simulink model "TorqueVect"  (R2022a)
settings: Solver=VariableStepAuto  StartTime=0.0  StopTime=32  RelTol=1e-3
PreLoadFcn:
  | run('Parameters\FSE_Parameters.m')
undefined symbols (not defined in the file): BRegenEnabledButton, canChannel, CyalphaLookUp, efficiency, Fz_curve, Fz_scaling_long, gearR, izz, jw, Kd, kd, Ki, ki, Kp, kp, l_f, l_r, lambda, m, Mz_max, N, N_lat, N_long, P_max, pid_kd_lat, pid_kd_long, pid_ki_lat, pid_ki_long, pid_kp_lat, pid_kp_long, R_max, rw, steerR, T_i_max, TC_Decr_Gas, TC_Derivative, TC_Incr_Gas, TC_On, TC_Relay_Off, TC_Relay_On, tireCornerStiffness, Ts, TV_On, TV_Override, velocity_lookup, velocity_lookup_lat, y_ref, yrr_scaling
libraries: simulink x218, slpidlib x135, CarMaker4SL x101, TractionControlLibrary x13, canmsglib x9, canlib x8, TorqueVectoringLibrary x6, simulink_extras x4, PedalConversionLibrary x3, PowerControlLibrary x1
(part 12 of 26)

== system TorqueVect/CarMaker/IPG Vehicle/PowerTrain/PTControl Example/PTControl_TV_MFE2/New TC/TC R2 ==
  modified slip ratio reference : Inport
  lim 1 : Inport  Port=2
  modified slip ratio measurement : Inport  Port=3
  P_TC : Inport  Port=4
  D_TC : Inport  Port=5
  enable_tc : Inport  Port=6
  PID Controller : slpidlib/PID Controller  Commented=on  Controller=PD  Form=Parallel  TimeDomain=Discrete-time  UseExternalTs=off  SampleTime=-1  IntegratorMethod=Forward Euler  FilterMethod=Forward Euler  ControllerParametersSource=external  P=125  I=1  UseKiTs=on  D=0  N=100  UseFilter=on  TunerSelectOption=Transfer Function Based (PID Tuner App)  InitialConditionSource=internal  InitialConditionForIntegrator=0  InitialConditionForFilter=0  DifferentiatorICPrevScaledInput=0  ExternalReset=none  TrackingMode=off  Kt=1  LimitOutput=on  SatLimitsSource=external  UpperSaturationLimit=inf  LowerSaturationLimit=-inf  LinearizeAsGain=on  AntiWindupMode=clamping  Kb=1  POutMin=[]  POutMax=[]  IOutMin=[]  IOutMax=[]  DOutMin=[]  DOutMax=[]  NOutMin=[]  NOutMax=[]  SumOutMin=[]  SumOutMax=[]  SaturationOutMin=[]  SaturationOutMax=[]  PParamMin=[]  PParamMax=[]  IParamMin=[]  IParamMax=[]  DParamMin=[]  DParamMax=[]  NParamMin=[]  NParamMax=[]  KbParamMin=[]  KbParamMax=[]  KtParamMin=[]  KtParamMax=[]  KbOutMin=[]  KbOutMax=[]  KtOutMin=[]  KtOutMax=[]  IntegratorOutMin=[]  IntegratorOutMax=[]  FilterOutMin=[]  FilterOutMax=[]  SumI1OutMin=[]  SumI1OutMax=[]  SumI2OutMin=[]  SumI2OutMax=[]  SumI3OutMin=[]  SumI3OutMax=[]  SumI4OutMin=[]  SumI4OutMax=[]  SumDOutMin=[]  SumDOutMax=[]  DifferentiatorOutMin=[]  DifferentiatorOutMax=[]  FilterDiffOutCoefMin=[]  FilterDiffOutCoefMax=[]  ReciprocalOutMin=[]  ReciprocalOutMax=[]  SumDenOutMin=[]  SumDenOutMax=[]  SumNumOutMin=[]  SumNumOutMax=[]  DivideOutMin=[]  DivideOutMax=[]  UdiffTsProdOutMin=[]  UdiffTsProdOutMax=[]  NTsProdOutMin=[]  NTsProdOutMax=[]  UintegralTsProdOutMin=[]  UintegralTsProdOutMax=[]  UngainTsProdOutMin=[]  UngainTsProdOutMax=[]  ClampingZeroOutDataTypeStr=Inherit: Inherit via back propagation  ClampingZeroOutMin=[]  ClampingZeroOutMax=[]  FilterDenConstantOutDataTypeStr=Inherit: Inherit via back propagation  FilterDenConstantOutMin=[]  FilterDenConstantOutMax=[]  PCopyOutDataTypeStr=Inherit: Inherit via back propagation  PCopyOutMin=[]  PCopyOutMax=[]  NCopyOutDataTypeStr=Inherit: Inherit via back propagation  NCopyOutMin=[]  NCopyOutMax=[]  IntegratorContinuousStateAttributes=''  IntegratorStateMustResolveToSignalObject=off  IntegratorRTWStateStorageClass=Auto  FilterContinuousStateAttributes=''  FilterStateMustResolveToSignalObject=off  FilterRTWStateStorageClass=Auto  ParallelPVariant=ExternalParameters  IdealPVariant=Disabled  IVariant=Disabled  DVariant=ExternalParameters  IntegratorVariant=Disabled  SatVariant=External  AWVariant=Disabled  PCopyVariant=Disabled  TRVariant=Disabled  FdbkBlocksVariant=Forward  IdealPFdbkVariant=Disabled  SatFdbkVariant=Disabled  DerivativeFilterVariant=ForwardEulerFilter  NVariant=ExternalParameters  NCopyVariant=Disabled  FilterICVariant=InternalICsFilter  IntegratorICVariant=Disabled  ExternalResetVariant=Disabled  TRSumVariant=Passthrough  SumFdbkVariant=Disabled  SumVariant=Sum_PD  TsampFilterVariant=InternalTs  TsampNgainVariant=Passthrough  TsampIntegralVariant=Disabled_SignalSpec  ExternalSaturationOutDataTypeStr=Inherit: Same as second input  aMode=0
  Sum1 : Sum  Inputs=|-+
  Sum2 : Sum  Commented=on  Inputs=|-+
  traction_controller : Subsystem
  Control Effort 1 : Outport
  wires:
  modified slip ratio reference/1 -> Sum1/1
  modified slip ratio measurement/1 -> Sum1/2
  lim 1/1 -> Sum2/2, traction_controller/1(max_torque)
  PID Controller/1 -> Sum2/1
  traction_controller/1(delta_torque) -> Control Effort 1/1
  enable_tc/1 -> traction_controller/3(enable_tc)
  Sum1/1 -> traction_controller/2(dslip)
  P_TC/1 -> traction_controller/4(Kp)
  D_TC/1 -> traction_controller/5(Kd)

== system TorqueVect/CarMaker/IPG Vehicle/PowerTrain/PTControl Example/PTControl_TV_MFE2/New TC/TC R3 ==
  modified slip ratio reference : Inport
  lim 1 : Inport  Port=2
  modified slip ratio measurement : Inport  Port=3
  P_TC : Inport  Port=4
  D_TC : Inport  Port=5
  enable_tc : Inport  Port=6
  PID Controller : slpidlib/PID Controller  Commented=on  Controller=PD  Form=Parallel  TimeDomain=Discrete-time  UseExternalTs=off  SampleTime=-1  IntegratorMethod=Forward Euler  FilterMethod=Forward Euler  ControllerParametersSource=external  P=125  I=1  UseKiTs=on  D=0  N=100  UseFilter=on  TunerSelectOption=Transfer Function Based (PID Tuner App)  InitialConditionSource=internal  InitialConditionForIntegrator=0  InitialConditionForFilter=0  DifferentiatorICPrevScaledInput=0  ExternalReset=none  TrackingMode=off  Kt=1  LimitOutput=on  SatLimitsSource=external  UpperSaturationLimit=inf  LowerSaturationLimit=-inf  LinearizeAsGain=on  AntiWindupMode=clamping  Kb=1  POutMin=[]  POutMax=[]  IOutMin=[]  IOutMax=[]  DOutMin=[]  DOutMax=[]  NOutMin=[]  NOutMax=[]  SumOutMin=[]  SumOutMax=[]  SaturationOutMin=[]  SaturationOutMax=[]  PParamMin=[]  PParamMax=[]  IParamMin=[]  IParamMax=[]  DParamMin=[]  DParamMax=[]  NParamMin=[]  NParamMax=[]  KbParamMin=[]  KbParamMax=[]  KtParamMin=[]  KtParamMax=[]  KbOutMin=[]  KbOutMax=[]  KtOutMin=[]  KtOutMax=[]  IntegratorOutMin=[]  IntegratorOutMax=[]  FilterOutMin=[]  FilterOutMax=[]  SumI1OutMin=[]  SumI1OutMax=[]  SumI2OutMin=[]  SumI2OutMax=[]  SumI3OutMin=[]  SumI3OutMax=[]  SumI4OutMin=[]  SumI4OutMax=[]  SumDOutMin=[]  SumDOutMax=[]  DifferentiatorOutMin=[]  DifferentiatorOutMax=[]  FilterDiffOutCoefMin=[]  FilterDiffOutCoefMax=[]  ReciprocalOutMin=[]  ReciprocalOutMax=[]  SumDenOutMin=[]  SumDenOutMax=[]  SumNumOutMin=[]  SumNumOutMax=[]  DivideOutMin=[]  DivideOutMax=[]  UdiffTsProdOutMin=[]  UdiffTsProdOutMax=[]  NTsProdOutMin=[]  NTsProdOutMax=[]  UintegralTsProdOutMin=[]  UintegralTsProdOutMax=[]  UngainTsProdOutMin=[]  UngainTsProdOutMax=[]  ClampingZeroOutDataTypeStr=Inherit: Inherit via back propagation  ClampingZeroOutMin=[]  ClampingZeroOutMax=[]  FilterDenConstantOutDataTypeStr=Inherit: Inherit via back propagation  FilterDenConstantOutMin=[]  FilterDenConstantOutMax=[]  PCopyOutDataTypeStr=Inherit: Inherit via back propagation  PCopyOutMin=[]  PCopyOutMax=[]  NCopyOutDataTypeStr=Inherit: Inherit via back propagation  NCopyOutMin=[]  NCopyOutMax=[]  IntegratorContinuousStateAttributes=''  IntegratorStateMustResolveToSignalObject=off  IntegratorRTWStateStorageClass=Auto  FilterContinuousStateAttributes=''  FilterStateMustResolveToSignalObject=off  FilterRTWStateStorageClass=Auto  ParallelPVariant=ExternalParameters  IdealPVariant=Disabled  IVariant=Disabled  DVariant=ExternalParameters  IntegratorVariant=Disabled  SatVariant=External  AWVariant=Disabled  PCopyVariant=Disabled  TRVariant=Disabled  FdbkBlocksVariant=Forward  IdealPFdbkVariant=Disabled  SatFdbkVariant=Disabled  DerivativeFilterVariant=ForwardEulerFilter  NVariant=ExternalParameters  NCopyVariant=Disabled  FilterICVariant=InternalICsFilter  IntegratorICVariant=Disabled  ExternalResetVariant=Disabled  TRSumVariant=Passthrough  SumFdbkVariant=Disabled  SumVariant=Sum_PD  TsampFilterVariant=InternalTs  TsampNgainVariant=Passthrough  TsampIntegralVariant=Disabled_SignalSpec  ExternalSaturationOutDataTypeStr=Inherit: Same as second input  aMode=0
  Sum1 : Sum  Inputs=|-+
  Sum2 : Sum  Commented=on  Inputs=|-+
  traction_controller : Subsystem
  Control Effort 1 : Outport
  wires:
  modified slip ratio reference/1 -> Sum1/1
  modified slip ratio measurement/1 -> Sum1/2
  lim 1/1 -> Sum2/2, traction_controller/1(max_torque)
  PID Controller/1 -> Sum2/1
  traction_controller/1(delta_torque) -> Control Effort 1/1
  enable_tc/1 -> traction_controller/3(enable_tc)
  Sum1/1 -> traction_controller/2(dslip)
  P_TC/1 -> traction_controller/4(Kp)
  D_TC/1 -> traction_controller/5(Kd)

== system TorqueVect/CarMaker/IPG Vehicle/PowerTrain/PTControl Example/PTControl_TV_MFE2/New TC/TC R4 ==
  modified slip ratio reference : Inport
  lim 1 : Inport  Port=2
  modified slip ratio measurement : Inport  Port=3
  P_TC : Inport  Port=4
  D_TC : Inport  Port=5
  enable_tc : Inport  Port=6
  PID Controller : slpidlib/PID Controller  Commented=on  Controller=PD  Form=Parallel  TimeDomain=Discrete-time  UseExternalTs=off  SampleTime=-1  IntegratorMethod=Forward Euler  FilterMethod=Forward Euler  ControllerParametersSource=external  P=125  I=1  UseKiTs=on  D=0  N=100  UseFilter=on  TunerSelectOption=Transfer Function Based (PID Tuner App)  InitialConditionSource=internal  InitialConditionForIntegrator=0  InitialConditionForFilter=0  DifferentiatorICPrevScaledInput=0  ExternalReset=none  TrackingMode=off  Kt=1  LimitOutput=on  SatLimitsSource=external  UpperSaturationLimit=inf  LowerSaturationLimit=-inf  LinearizeAsGain=on  AntiWindupMode=clamping  Kb=1  POutMin=[]  POutMax=[]  IOutMin=[]  IOutMax=[]  DOutMin=[]  DOutMax=[]  NOutMin=[]  NOutMax=[]  SumOutMin=[]  SumOutMax=[]  SaturationOutMin=[]  SaturationOutMax=[]  PParamMin=[]  PParamMax=[]  IParamMin=[]  IParamMax=[]  DParamMin=[]  DParamMax=[]  NParamMin=[]  NParamMax=[]  KbParamMin=[]  KbParamMax=[]  KtParamMin=[]  KtParamMax=[]  KbOutMin=[]  KbOutMax=[]  KtOutMin=[]  KtOutMax=[]  IntegratorOutMin=[]  IntegratorOutMax=[]  FilterOutMin=[]  FilterOutMax=[]  SumI1OutMin=[]  SumI1OutMax=[]  SumI2OutMin=[]  SumI2OutMax=[]  SumI3OutMin=[]  SumI3OutMax=[]  SumI4OutMin=[]  SumI4OutMax=[]  SumDOutMin=[]  SumDOutMax=[]  DifferentiatorOutMin=[]  DifferentiatorOutMax=[]  FilterDiffOutCoefMin=[]  FilterDiffOutCoefMax=[]  ReciprocalOutMin=[]  ReciprocalOutMax=[]  SumDenOutMin=[]  SumDenOutMax=[]  SumNumOutMin=[]  SumNumOutMax=[]  DivideOutMin=[]  DivideOutMax=[]  UdiffTsProdOutMin=[]  UdiffTsProdOutMax=[]  NTsProdOutMin=[]  NTsProdOutMax=[]  UintegralTsProdOutMin=[]  UintegralTsProdOutMax=[]  UngainTsProdOutMin=[]  UngainTsProdOutMax=[]  ClampingZeroOutDataTypeStr=Inherit: Inherit via back propagation  ClampingZeroOutMin=[]  ClampingZeroOutMax=[]  FilterDenConstantOutDataTypeStr=Inherit: Inherit via back propagation  FilterDenConstantOutMin=[]  FilterDenConstantOutMax=[]  PCopyOutDataTypeStr=Inherit: Inherit via back propagation  PCopyOutMin=[]  PCopyOutMax=[]  NCopyOutDataTypeStr=Inherit: Inherit via back propagation  NCopyOutMin=[]  NCopyOutMax=[]  IntegratorContinuousStateAttributes=''  IntegratorStateMustResolveToSignalObject=off  IntegratorRTWStateStorageClass=Auto  FilterContinuousStateAttributes=''  FilterStateMustResolveToSignalObject=off  FilterRTWStateStorageClass=Auto  ParallelPVariant=ExternalParameters  IdealPVariant=Disabled  IVariant=Disabled  DVariant=ExternalParameters  IntegratorVariant=Disabled  SatVariant=External  AWVariant=Disabled  PCopyVariant=Disabled  TRVariant=Disabled  FdbkBlocksVariant=Forward  IdealPFdbkVariant=Disabled  SatFdbkVariant=Disabled  DerivativeFilterVariant=ForwardEulerFilter  NVariant=ExternalParameters  NCopyVariant=Disabled  FilterICVariant=InternalICsFilter  IntegratorICVariant=Disabled  ExternalResetVariant=Disabled  TRSumVariant=Passthrough  SumFdbkVariant=Disabled  SumVariant=Sum_PD  TsampFilterVariant=InternalTs  TsampNgainVariant=Passthrough  TsampIntegralVariant=Disabled_SignalSpec  ExternalSaturationOutDataTypeStr=Inherit: Same as second input  aMode=0
  Sum1 : Sum  Inputs=|-+
  Sum2 : Sum  Commented=on  Inputs=|-+
  traction_controller : Subsystem
  Control Effort 1 : Outport
  wires:
  modified slip ratio reference/1 -> Sum1/1
  modified slip ratio measurement/1 -> Sum1/2
  lim 1/1 -> Sum2/2, traction_controller/1(max_torque)
  PID Controller/1 -> Sum2/1
  traction_controller/1(delta_torque) -> Control Effort 1/1
  enable_tc/1 -> traction_controller/3(enable_tc)
  Sum1/1 -> traction_controller/2(dslip)
  P_TC/1 -> traction_controller/4(Kp)
  D_TC/1 -> traction_controller/5(Kd)

== system TorqueVect/CarMaker/IPG Vehicle/PowerTrain/PTControl Example/PTControl_TV_MFE2/Subsystem/PedalConversion ==
  rThrottlePedal : Inport  OutMin=0  OutMax=1  PortDimensions=1
      settings: AttributesFormatString=[%<OutMin>, %<OutMax>]
  Pedal Mapping w/Regen : Lookup_n-D  NumberOfTableDimensions=1  BreakpointsForDimension1=[0 0.08 0.1 1]  Table=[-1 0 0 1]  InternalRulePriority=Speed  OutMin=-1  OutMax=1  RndMeth=Simplest
  Saturation : Saturate  UpperLimit=1  LowerLimit=-1  OutMin=-1  OutMax=1
      settings: AttributesFormatString=[%<LowerLimit>, %<UpperLimit>]
  rThrottle : Outport  OutMin=-1  OutMax=1
      settings: AttributesFormatString=[%<OutMin>, %<OutMax>]
  wires:
  Saturation/1 -> rThrottle/1
  Pedal Mapping w/Regen/1 -> Saturation/1
  rThrottlePedal/1 -> Pedal Mapping w/Regen/1

== system TorqueVect/CarMaker/IPG Vehicle/PowerTrain/PTControl Example/PTControl_TV_MFE2/Subsystem/Subsystem ==
  vLat : Inport  Unit=m/s  PortDimensions=1
      settings: AttributesFormatString=%<Unit>
  vLong : Inport  Port=2  Unit=m/s  PortDimensions=1
      settings: AttributesFormatString=%<Unit>
  aSteerWheel : Inport  Port=3  Unit=rad  PortDimensions=1
      settings: AttributesFormatString=%<Unit>
  rSteerWheel : Inport  Port=4
  Add1 : Sum  Inputs=-+
  Atan : Trigonometry  Operator=atan
  Divide : Product  Inputs=*/
  Gain : Gain  Gain=-1
  Product : Product
  Saturation : Saturate  UpperLimit=60  LowerLimit=1
  aSlip : Outport  VectorParamsAs1DForOutWhenUnconnected=off
  wires:
  rSteerWheel/1 -> Product/2
  vLong/1 -> Saturation/1
  vLat/1 -> Divide/1
  Product/1 -> Add1/2  "Wheel Angle"
  Atan/1 -> Add1/1  "Yaw Angle"
  Gain/1 -> aSlip/1
  aSteerWheel/1 -> Product/1
  Saturation/1 -> Divide/2
  Divide/1 -> Atan/1
  Add1/1 -> Gain/1  "Error"

== system TorqueVect/CarMaker/IPG Vehicle/PowerTrain/PTControl Example/PTControl_TV_MFE2/Subsystem/TV Enable Checker ==
  vLong : Inport  Unit=m/s  PortDimensions=1
      settings: AttributesFormatString=%<Unit>
  aSteerWheel : Inport  Port=2  Unit=rad  PortDimensions=1
      settings: AttributesFormatString=%<Unit>
  vLongMin : Inport  Port=3  Unit=m/s  PortDimensions=1
      settings: AttributesFormatString=%<Unit>
  aSteerWheelMin : Inport  Port=4  Unit=rad  PortDimensions=1
      settings: AttributesFormatString=%<Unit>
  BTorqueVectoringEnable : Inport  Port=5
  Abs : Abs  ZeroCross=off  SaturateOnIntegerOverflow=off
  Logical Operator : Logic  Inputs=3  AllPortsSameDT=off  OutDataTypeStr=boolean
  Relational Operator : RelationalOperator  Operator=>  OutDataTypeStr=boolean  RndMeth=Simplest  InputSameDT=off
  Relational Operator1 : RelationalOperator  Operator=>  OutDataTypeStr=boolean  RndMeth=Simplest  InputSameDT=off
  BEnable : Outport  VectorParamsAs1DForOutWhenUnconnected=off
  wires:
  Relational Operator1/1 -> Logical Operator/2
  vLongMin/1 -> Relational Operator/2
  Logical Operator/1 -> BEnable/1
  Relational Operator/1 -> Logical Operator/1
  vLong/1 -> Relational Operator/1
  BTorqueVectoringEnable/1 -> Logical Operator/3
  Abs/1 -> Relational Operator1/1
  aSteerWheelMin/1 -> Relational Operator1/2
  aSteerWheel/1 -> Abs/1

== system TorqueVect/CarMaker/IPG Vehicle/PowerTrain/PTControl Example/PTControl_TV_MFE2/Subsystem/TorqueSplit ==
  rSplitF : Inport
  rThrottle : Inport  Port=2
  MMotorMax : Inport  Port=3
  MRegenMotorMax : Inport  Port=4
  Add : Sum  Inputs=-+
  Gain : Gain  Gain=4
  MATLAB Function : MATLAB Function  TreatAsAtomicUnit=on
  Product : Product
  Product1 : Product
  Switch : Switch  Criteria=u2 > Threshold  SaturateOnIntegerOverflow=off  InputSameDT=off
  MMotorDemandFL : Outport
  MMotorDemandFR : Outport  Port=2
  MMotorDemandRL : Outport  Port=3
  MMotorDemandRR : Outport  Port=4
  wires:
  MATLAB Function/4(rr_out) -> MMotorDemandRR/1
  MATLAB Function/3(rl_out) -> MMotorDemandRL/1
  Product1/1 -> MATLAB Function/1(f_in), Add/1
  rSplitF/1 -> Product1/1
  MATLAB Function/2(fr_out) -> MMotorDemandFR/1
  MATLAB Function/1(fl_out) -> MMotorDemandFL/1
  Product/1 -> Add/2, Product1/2
  Add/1 -> MATLAB Function/2(r_in)
  rThrottle/1 -> Switch/2, Product/2
  MMotorMax/1 -> Switch/1
  Gain/1 -> Product/1
  Switch/1 -> MATLAB Function/3(maxTrq), Gain/1
  MRegenMotorMax/1 -> Switch/3

== system TorqueVect/CarMaker/IPG Vehicle/PowerTrain/PTControl Example/PTControl_TV_MFE2/Subsystem/TorqueVectoringAlgorithm ==
  BEnable : Inport
  NTorqueMaxDelta : Inport  Port=2
  NTorqueMax : Inport  Port=3
  NTorqueAxle : Inport  Port=4
  aSlip : Inport  Port=5
  P_YR : Inport  Port=6
  D_YR : Inport  Port=7
  NBrake : Inport  Port=8
  Abs : Abs  SaturateOnIntegerOverflow=off
  Abs2 : Abs  SaturateOnIntegerOverflow=off
  Add : Sum  Inputs=+-
  Gain : Gain  Gain=0.5
  Gain1 : Gain  Gain=-1
  If : If  IfExpression=u1 < 0.4
  If Action Subsystem : Subsystem  TreatAsAtomicUnit=on
  If Action Subsystem1 : Subsystem  TreatAsAtomicUnit=on
  Merge : Merge
  Merge1 : Merge
  Min : MinMax  Inputs=3
  PID Controller : slpidlib/PID Controller  Controller=PD  Form=Parallel  TimeDomain=Continuous-time  UseExternalTs=off  SampleTime=-1  IntegratorMethod=Forward Euler  FilterMethod=Forward Euler  ControllerParametersSource=external  P=1  I=1  UseKiTs=off  D=0  N=100  UseFilter=on  TunerSelectOption=Transfer Function Based (PID Tuner App)  InitialConditionSource=internal  InitialConditionForIntegrator=0  InitialConditionForFilter=0  DifferentiatorICPrevScaledInput=0  ExternalReset=either  TrackingMode=off  Kt=1  LimitOutput=off  SatLimitsSource=internal  UpperSaturationLimit=inf  LowerSaturationLimit=-inf  LinearizeAsGain=on  AntiWindupMode=none  Kb=1  POutMin=[]  POutMax=[]  IOutMin=[]  IOutMax=[]  DOutMin=[]  DOutMax=[]  NOutMin=[]  NOutMax=[]  SumOutMin=[]  SumOutMax=[]  SaturationOutMin=[]  SaturationOutMax=[]  PParamMin=[]  PParamMax=[]  IParamMin=[]  IParamMax=[]  DParamMin=[]  DParamMax=[]  NParamMin=[]  NParamMax=[]  KbParamMin=[]  KbParamMax=[]  KtParamMin=[]  KtParamMax=[]  KbOutMin=[]  KbOutMax=[]  KtOutMin=[]  KtOutMax=[]  IntegratorOutMin=[]  IntegratorOutMax=[]  FilterOutMin=[]  FilterOutMax=[]  SumI1OutMin=[]  SumI1OutMax=[]  SumI2OutMin=[]  SumI2OutMax=[]  SumI3OutMin=[]  SumI3OutMax=[]  SumI4OutMin=[]  SumI4OutMax=[]  SumDOutMin=[]  SumDOutMax=[]  DifferentiatorOutMin=[]  DifferentiatorOutMax=[]  FilterDiffOutCoefMin=[]  FilterDiffOutCoefMax=[]  ReciprocalOutMin=[]  ReciprocalOutMax=[]  SumDenOutMin=[]  SumDenOutMax=[]  SumNumOutMin=[]  SumNumOutMax=[]  DivideOutMin=[]  DivideOutMax=[]  UdiffTsProdOutMin=[]  UdiffTsProdOutMax=[]  NTsProdOutMin=[]  NTsProdOutMax=[]  UintegralTsProdOutMin=[]  UintegralTsProdOutMax=[]  UngainTsProdOutMin=[]  UngainTsProdOutMax=[]  ClampingZeroOutDataTypeStr=Inherit: Inherit via back propagation  ClampingZeroOutMin=[]  ClampingZeroOutMax=[]  FilterDenConstantOutDataTypeStr=Inherit: Inherit via back propagation  FilterDenConstantOutMin=[]  FilterDenConstantOutMax=[]  PCopyOutDataTypeStr=Inherit: Inherit via back propagation  PCopyOutMin=[]  PCopyOutMax=[]  NCopyOutDataTypeStr=Inherit: Inherit via back propagation  NCopyOutMin=[]  NCopyOutMax=[]  IntegratorContinuousStateAttributes=''  IntegratorStateMustResolveToSignalObject=off  IntegratorRTWStateStorageClass=Auto  FilterContinuousStateAttributes=''  FilterStateMustResolveToSignalObject=off  FilterRTWStateStorageClass=Auto  ParallelPVariant=ExternalParameters  IdealPVariant=Disabled  IVariant=Disabled  DVariant=ExternalParameters  IntegratorVariant=Disabled  SatVariant=Disabled  AWVariant=Disabled  PCopyVariant=Disabled  TRVariant=Disabled  FdbkBlocksVariant=Forward  IdealPFdbkVariant=Disabled  SatFdbkVariant=Disabled  DerivativeFilterVariant=ContFilter  NVariant=ExternalParameters  NCopyVariant=Disabled  FilterICVariant=InternalICsFilter  IntegratorICVariant=Disabled  ExternalResetVariant=ExternalReset  TRSumVariant=Passthrough  SumFdbkVariant=Disabled  SumVariant=Sum_PD  TsampFilterVariant=InternalTs  TsampNgainVariant=Passthrough  TsampIntegralVariant=Disabled_SignalSpec  ExternalSaturationOutDataTypeStr=Inherit: Same as second input  aMode=0
  Product : Product  Inputs=3
  Saturation Dynamic : simulink/Discontinuities/Saturation Dynamic  OutMin=[]  OutMax=[]  OutDataTypeStr=Inherit: Same as second input  OutDataType=fixdt(1, 16)  OutScaling=2^-10  DoSatur=off
  Saturation Dynamic1 : simulink/Discontinuities/Saturation Dynamic  OutMin=[]  OutMax=[]  OutDataTypeStr=Inherit: Same as second input  OutDataType=fixdt(1, 16)  OutScaling=2^-10  DoSatur=off
  Sign : Signum
  NTorqueLeftOut : Outport
  NTorqueRightOut : Outport  Port=2
  wires:
  Gain1/1 -> Saturation Dynamic1/3, Saturation Dynamic/3
  Merge/1 -> Saturation Dynamic1/2
  Saturation Dynamic1/1 -> NTorqueRightOut/1
  [NTorqueMax] -> Gain1/1, Saturation Dynamic1/1, Saturation Dynamic/1
  Saturation Dynamic/1 -> NTorqueLeftOut/1
  Merge1/1 -> Saturation Dynamic/2
  [NTorqueMax] -> Add/1
  NTorqueMax/1 -> [NTorqueMax]
  Gain/1 -> [NTorqueWheel]
  NTorqueAxle/1 -> Gain/1
  [BEnable] -> PID Controller/5
  [BEnable] -> Product/1
  BEnable/1 -> [BEnable]
  [NTorqueWheel] -> Abs/1
  Sign/1 -> Product/3
  If Action Subsystem1/2(NTorqueRightOut) -> Merge/2
  If Action Subsystem1/1(NTorqueLeftOut) -> Merge1/2
  Product/1 -> If Action Subsystem/2(NTorqueDelta)
  Add/1 -> Min/2
  [NTorqueWheel] -> If Action Subsystem/1(NTorqueWheel), If Action Subsystem1/2(NTorqueWheel1), If Action Subsystem1/1(NTorqueWheel)
  aSlip/1 -> PID Controller/1
  Abs/1 -> Add/2
  D_YR/1 -> PID Controller/3
  P_YR/1 -> PID Controller/2
  If Action Subsystem/1(NTorqueLeftOut) -> Merge1/1
  PID Controller/1 -> [NTorqueTV]
  [NTorqueTV] -> Abs2/1
  NTorqueMaxDelta/1 -> Min/1
  Abs2/1 -> Min/3
  If/1 -> If Action Subsystem/Action
  If Action Subsystem/2(NTorqueRightOut) -> Merge/1
  [NTorqueTV] -> Sign/1
  NBrake/1 -> If/1
  If/2 -> If Action Subsystem1/Action
  Min/1 -> Product/2

== system TorqueVect/CarMaker/IPG Vehicle/PowerTrain/PTControl Example/PTControl_TV_MFE2/Subsystem/TorqueVectoringAlgorithm1 ==
  BEnable : Inport
  NTorqueMaxDelta : Inport  Port=2
  NTorqueMax : Inport  Port=3
  NTorqueAxle : Inport  Port=4
  aSlip : Inport  Port=5
  P_YR : Inport  Port=6
  D_YR : Inport  Port=7
  NBrake : Inport  Port=8
  Abs : Abs  SaturateOnIntegerOverflow=off
  Abs2 : Abs  SaturateOnIntegerOverflow=off
  Add : Sum  Inputs=+-
  Gain : Gain  Gain=0.5
  Gain1 : Gain  Gain=-1
  If : If  IfExpression=u1 < 0.4
  If Action Subsystem : Subsystem  TreatAsAtomicUnit=on
  If Action Subsystem1 : Subsystem  TreatAsAtomicUnit=on
  Merge : Merge
  Merge1 : Merge
  Min : MinMax  Inputs=3
  PID Controller : slpidlib/PID Controller  Controller=PD  Form=Parallel  TimeDomain=Continuous-time  UseExternalTs=off  SampleTime=-1  IntegratorMethod=Forward Euler  FilterMethod=Forward Euler  ControllerParametersSource=external  P=1  I=1  UseKiTs=off  D=0  N=100  UseFilter=on  TunerSelectOption=Transfer Function Based (PID Tuner App)  InitialConditionSource=internal  InitialConditionForIntegrator=0  InitialConditionForFilter=0  DifferentiatorICPrevScaledInput=0  ExternalReset=either  TrackingMode=off  Kt=1  LimitOutput=off  SatLimitsSource=internal  UpperSaturationLimit=inf  LowerSaturationLimit=-inf  LinearizeAsGain=on  AntiWindupMode=none  Kb=1  POutMin=[]  POutMax=[]  IOutMin=[]  IOutMax=[]  DOutMin=[]  DOutMax=[]  NOutMin=[]  NOutMax=[]  SumOutMin=[]  SumOutMax=[]  SaturationOutMin=[]  SaturationOutMax=[]  PParamMin=[]  PParamMax=[]  IParamMin=[]  IParamMax=[]  DParamMin=[]  DParamMax=[]  NParamMin=[]  NParamMax=[]  KbParamMin=[]  KbParamMax=[]  KtParamMin=[]  KtParamMax=[]  KbOutMin=[]  KbOutMax=[]  KtOutMin=[]  KtOutMax=[]  IntegratorOutMin=[]  IntegratorOutMax=[]  FilterOutMin=[]  FilterOutMax=[]  SumI1OutMin=[]  SumI1OutMax=[]  SumI2OutMin=[]  SumI2OutMax=[]  SumI3OutMin=[]  SumI3OutMax=[]  SumI4OutMin=[]  SumI4OutMax=[]  SumDOutMin=[]  SumDOutMax=[]  DifferentiatorOutMin=[]  DifferentiatorOutMax=[]  FilterDiffOutCoefMin=[]  FilterDiffOutCoefMax=[]  ReciprocalOutMin=[]  ReciprocalOutMax=[]  SumDenOutMin=[]  SumDenOutMax=[]  SumNumOutMin=[]  SumNumOutMax=[]  DivideOutMin=[]  DivideOutMax=[]  UdiffTsProdOutMin=[]  UdiffTsProdOutMax=[]  NTsProdOutMin=[]  NTsProdOutMax=[]  UintegralTsProdOutMin=[]  UintegralTsProdOutMax=[]  UngainTsProdOutMin=[]  UngainTsProdOutMax=[]  ClampingZeroOutDataTypeStr=Inherit: Inherit via back propagation  ClampingZeroOutMin=[]  ClampingZeroOutMax=[]  FilterDenConstantOutDataTypeStr=Inherit: Inherit via back propagation  FilterDenConstantOutMin=[]  FilterDenConstantOutMax=[]  PCopyOutDataTypeStr=Inherit: Inherit via back propagation  PCopyOutMin=[]  PCopyOutMax=[]  NCopyOutDataTypeStr=Inherit: Inherit via back propagation  NCopyOutMin=[]  NCopyOutMax=[]  IntegratorContinuousStateAttributes=''  IntegratorStateMustResolveToSignalObject=off  IntegratorRTWStateStorageClass=Auto  FilterContinuousStateAttributes=''  FilterStateMustResolveToSignalObject=off  FilterRTWStateStorageClass=Auto  ParallelPVariant=ExternalParameters  IdealPVariant=Disabled  IVariant=Disabled  DVariant=ExternalParameters  IntegratorVariant=Disabled  SatVariant=Disabled  AWVariant=Disabled  PCopyVariant=Disabled  TRVariant=Disabled  FdbkBlocksVariant=Forward  IdealPFdbkVariant=Disabled  SatFdbkVariant=Disabled  DerivativeFilterVariant=ContFilter  NVariant=ExternalParameters  NCopyVariant=Disabled  FilterICVariant=InternalICsFilter  IntegratorICVariant=Disabled  ExternalResetVariant=ExternalReset  TRSumVariant=Passthrough  SumFdbkVariant=Disabled  SumVariant=Sum_PD  TsampFilterVariant=InternalTs  TsampNgainVariant=Passthrough  TsampIntegralVariant=Disabled_SignalSpec  ExternalSaturationOutDataTypeStr=Inherit: Same as second input  aMode=0
  Product : Product  Inputs=3
  Saturation Dynamic : simulink/Discontinuities/Saturation Dynamic  OutMin=[]  OutMax=[]  OutDataTypeStr=Inherit: Same as second input  OutDataType=fixdt(1, 16)  OutScaling=2^-10  DoSatur=off
  Saturation Dynamic1 : simulink/Discontinuities/Saturation Dynamic  OutMin=[]  OutMax=[]  OutDataTypeStr=Inherit: Same as second input  OutDataType=fixdt(1, 16)  OutScaling=2^-10  DoSatur=off
  Sign : Signum
  NTorqueLeftOut : Outport
  NTorqueRightOut : Outport  Port=2
  wires:
  Gain1/1 -> Saturation Dynamic1/3, Saturation Dynamic/3
  Merge/1 -> Saturation Dynamic1/2
  Saturation Dynamic1/1 -> NTorqueRightOut/1
  [NTorqueMax] -> Gain1/1, Saturation Dynamic1/1, Saturation Dynamic/1
  Saturation Dynamic/1 -> NTorqueLeftOut/1
  Merge1/1 -> Saturation Dynamic/2
  [NTorqueMax] -> Add/1
  NTorqueMax/1 -> [NTorqueMax]
  Gain/1 -> [NTorqueWheel]
  NTorqueAxle/1 -> Gain/1
  [BEnable] -> PID Controller/5
  [BEnable] -> Product/1
  BEnable/1 -> [BEnable]
  [NTorqueWheel] -> Abs/1
  Sign/1 -> Product/3
  If Action Subsystem1/2(NTorqueRightOut) -> Merge/2
  If Action Subsystem1/1(NTorqueLeftOut) -> Merge1/2
  Product/1 -> If Action Subsystem/2(NTorqueDelta)
  Add/1 -> Min/2
  [NTorqueWheel] -> If Action Subsystem/1(NTorqueWheel), If Action Subsystem1/2(NTorqueWheel1), If Action Subsystem1/1(NTorqueWheel)
  aSlip/1 -> PID Controller/1
  Abs/1 -> Add/2
  D_YR/1 -> PID Controller/3
  P_YR/1 -> PID Controller/2
  If Action Subsystem/1(NTorqueLeftOut) -> Merge1/1
  PID Controller/1 -> [NTorqueTV]
  [NTorqueTV] -> Abs2/1
  NTorqueMaxDelta/1 -> Min/1
  Abs2/1 -> Min/3
  If/1 -> If Action Subsystem/Action
  If Action Subsystem/2(NTorqueRightOut) -> Merge/1
  [NTorqueTV] -> Sign/1
  NBrake/1 -> If/1
  If/2 -> If Action Subsystem1/Action
  Min/1 -> Product/2

== system TorqueVect/CarMaker/IPG Vehicle/PowerTrain/PTControl Example/PTControl_TV_MFE25/Full Control Loop/Reference Generator ==
  note: 4 normal loads come in
  note: For throttle sign and Product:
      | If positive, normal reference
      | If negative (regen), similar reference but negative (negative target slip*times speed), this might need to change to account for regen limits
      | If 0, target zero
  note: select target slip ratio for each
  note: Manipulate to get target reference for each wheel
  note: Vehicle velocity
  note: Modified slip ratio targets
  u : Inport
  Fz_per_wheel : Inport  Port=2
  vehicle_speed : Inport  Port=3
  min_speed : Inport  Port=4
  1-D Lookup Table{,1..3} (4 alike) : Lookup_n-D  NumberOfTableDimensions=1  BreakpointsForDimension1Source=Input port  BreakpointsForDimension1=[-5:5]  TableSource=Input port  Table=tanh([-5:5])  InternalRulePriority=Speed  RndMeth=Simplest
      settings: InputPortMap=u0,p221,p5
  Constant : Constant  Value=y_ref
  Constant1 : Constant  Value=Fz_curve
  Demux1 : Demux
  Max : MinMax  Function=max  Inputs=2
  Product{,1..3} (4 alike) : Product  Inputs=3
  Throttle_Sign : Signum
  Y_Reference : MATLAB Function  Commented=on  TreatAsAtomicUnit=on
  r1 : Outport
  r2 : Outport  Port=2
  r3 : Outport  Port=3
  r4 : Outport  Port=4
  wires:
  Product1/1 -> r2/1
  Product2/1 -> r3/1
  Product3/1 -> r4/1
  u/1 -> Throttle_Sign/1
  Throttle_Sign/1 -> Product3/1, Product2/1, Product1/1, Product/1
  vehicle_speed/1 -> Max/1
  Demux1/1 -> 1-D Lookup Table/1
  Fz_per_wheel/1 -> Demux1/1
  Demux1/2 -> 1-D Lookup Table1/1
  Demux1/3 -> 1-D Lookup Table2/1
  Demux1/4 -> 1-D Lookup Table3/1
  1-D Lookup Table/1 -> Product/3  "Target kappa"
  1-D Lookup Table1/1 -> Product1/3  "Target kappa"
  1-D Lookup Table2/1 -> Product2/3  "Target kappa"
  1-D Lookup Table3/1 -> Product3/3  "Target kappa"
  Product/1 -> r1/1
  min_speed/1 -> Max/2
  Constant/1 -> 1-D Lookup Table3/2, 1-D Lookup Table2/2, 1-D Lookup Table1/2, 1-D Lookup Table/2
  Constant1/1 -> 1-D Lookup Table3/3, 1-D Lookup Table2/3, 1-D Lookup Table1/3, 1-D Lookup Table/3
  Max/1 -> Product3/2, Product1/2, Product/2, Product2/2  "Reference"

== system TorqueVect/CarMaker/IPG Vehicle/PowerTrain/PTControl Example/PTControl_TV_MFE25/Full Control Loop/TC 1 ==
  modified slip ratio reference : Inport
  u_lim : Inport  Port=2
  modified slip ratio measurement : Inport  Port=3
  l_lim : Inport  Port=4
  ResetSignal : Inport  Port=5
  velocity : Inport  Port=6
  Constant : Constant  Value=kp
  Constant1 : Constant  Value=ki
  Constant2 : Constant  Value=kd
  Constant3 : Constant  Value=N
  PID Controller : slpidlib/PID Controller  Controller=PID  Form=Parallel  TimeDomain=Discrete-time  UseExternalTs=off  SampleTime=Ts  IntegratorMethod=Trapezoidal  FilterMethod=Forward Euler  ControllerParametersSource=external  P=kp  I=ki  UseKiTs=on  D=kd  N=100  UseFilter=on  TunerSelectOption=Transfer Function Based (PID Tuner App)  InitialConditionSource=internal  InitialConditionForIntegrator=0  InitialConditionForFilter=0  DifferentiatorICPrevScaledInput=0  ExternalReset=either  TrackingMode=off  Kt=1  LimitOutput=on  SatLimitsSource=external  UpperSaturationLimit=inf  LowerSaturationLimit=-inf  LinearizeAsGain=on  AntiWindupMode=clamping  Kb=1  POutMin=[]  POutMax=[]  IOutMin=[]  IOutMax=[]  DOutMin=[]  DOutMax=[]  NOutMin=[]  NOutMax=[]  SumOutMin=[]  SumOutMax=[]  SaturationOutMin=[]  SaturationOutMax=[]  PParamMin=[]  PParamMax=[]  IParamMin=[]  IParamMax=[]  DParamMin=[]  DParamMax=[]  NParamMin=[]  NParamMax=[]  KbParamMin=[]  KbParamMax=[]  KtParamMin=[]  KtParamMax=[]  KbOutMin=[]  KbOutMax=[]  KtOutMin=[]  KtOutMax=[]  IntegratorOutMin=[]  IntegratorOutMax=[]  FilterOutMin=[]  FilterOutMax=[]  SumI1OutMin=[]  SumI1OutMax=[]  SumI2OutMin=[]  SumI2OutMax=[]  SumI3OutMin=[]  SumI3OutMax=[]  SumI4OutMin=[]  SumI4OutMax=[]  SumDOutMin=[]  SumDOutMax=[]  DifferentiatorOutMin=[]  DifferentiatorOutMax=[]  FilterDiffOutCoefMin=[]  FilterDiffOutCoefMax=[]  ReciprocalOutMin=[]  ReciprocalOutMax=[]  SumDenOutMin=[]  SumDenOutMax=[]  SumNumOutMin=[]  SumNumOutMax=[]  DivideOutMin=[]  DivideOutMax=[]  UdiffTsProdOutMin=[]  UdiffTsProdOutMax=[]  NTsProdOutMin=[]  NTsProdOutMax=[]  UintegralTsProdOutMin=[]  UintegralTsProdOutMax=[]  UngainTsProdOutMin=[]  UngainTsProdOutMax=[]  ClampingZeroOutDataTypeStr=Inherit: Inherit via back propagation  ClampingZeroOutMin=[]  ClampingZeroOutMax=[]  FilterDenConstantOutDataTypeStr=Inherit: Inherit via back propagation  FilterDenConstantOutMin=[]  FilterDenConstantOutMax=[]  PCopyOutDataTypeStr=Inherit: Inherit via back propagation  PCopyOutMin=[]  PCopyOutMax=[]  NCopyOutDataTypeStr=Inherit: Inherit via back propagation  NCopyOutMin=[]  NCopyOutMax=[]  IntegratorContinuousStateAttributes=''  IntegratorStateMustResolveToSignalObject=off  IntegratorRTWStateStorageClass=Auto  FilterContinuousStateAttributes=''  FilterStateMustResolveToSignalObject=off  FilterRTWStateStorageClass=Auto  ParallelPVariant=ExternalParameters  IdealPVariant=Disabled  IVariant=ExternalParameters  DVariant=ExternalParameters  IntegratorVariant=Discrete  SatVariant=External  AWVariant=DiscClampingParallel  PCopyVariant=Disabled  TRVariant=Disabled  FdbkBlocksVariant=Feedback  IdealPFdbkVariant=Passthrough  SatFdbkVariant=Passthrough  DerivativeFilterVariant=ForwardEulerFilter  NVariant=ExternalParameters  NCopyVariant=Disabled  FilterICVariant=InternalICsFilter  IntegratorICVariant=InternalICs  ExternalResetVariant=ExternalReset  TRSumVariant=Passthrough  SumFdbkVariant=Enabled  SumVariant=Sum_PID  TsampFilterVariant=InternalTs  TsampNgainVariant=Passthrough  TsampIntegralVariant=Passthrough  ExternalSaturationOutDataTypeStr=Inherit: Same as second input  aMode=0
  Subsystem : Subsystem
  Sum1 : Sum  Inputs=|+-
  velocity lookup : Constant  Value=velocity_lookup
  Control Effort 1 : Outport
  wires:
  Constant3/1 -> PID Controller/5
  Constant2/1 -> Subsystem/5(pid_kd)
  Constant1/1 -> Subsystem/4(pid_ki)
  Subsystem/3(Out3) -> PID Controller/4
  Subsystem/2(Out2) -> PID Controller/3
  Subsystem/1(Out1) -> PID Controller/2
  velocity lookup/1 -> Subsystem/3(velocity lookup)
  Constant/1 -> Subsystem/2(pid_kp)
  velocity/1 -> Subsystem/1(velocity)
  ResetSignal/1 -> PID Controller/6
  PID Controller/1 -> Control Effort 1/1
  l_lim/1 -> PID Controller/8
  modified slip ratio measurement/1 -> Sum1/2
  u_lim/1 -> PID Controller/7
  modified slip ratio reference/1 -> Sum1/1
  Sum1/1 -> PID Controller/1  "error 1"

== system TorqueVect/CarMaker/IPG Vehicle/PowerTrain/PTControl Example/PTControl_TV_MFE25/Full Control Loop/TC 2 ==
  modified slip ratio reference : Inport
  u_lim : Inport  Port=2
  modified slip ratio measurement : Inport  Port=3
  l_lim : Inport  Port=4
  ResetSignal : Inport  Port=5
  velocity : Inport  Port=6
  Constant : Constant  Value=kp
  Constant1 : Constant  Value=ki
  Constant2 : Constant  Value=kd
  Constant3 : Constant  Value=N
  PID Controller : slpidlib/PID Controller  Controller=PID  Form=Parallel  TimeDomain=Discrete-time  UseExternalTs=off  SampleTime=Ts  IntegratorMethod=Trapezoidal  FilterMethod=Forward Euler  ControllerParametersSource=external  P=kp  I=ki  UseKiTs=on  D=kd  N=100  UseFilter=on  TunerSelectOption=Transfer Function Based (PID Tuner App)  InitialConditionSource=internal  InitialConditionForIntegrator=0  InitialConditionForFilter=0  DifferentiatorICPrevScaledInput=0  ExternalReset=either  TrackingMode=off  Kt=1  LimitOutput=on  SatLimitsSource=external  UpperSaturationLimit=inf  LowerSaturationLimit=-inf  LinearizeAsGain=on  AntiWindupMode=clamping  Kb=1  POutMin=[]  POutMax=[]  IOutMin=[]  IOutMax=[]  DOutMin=[]  DOutMax=[]  NOutMin=[]  NOutMax=[]  SumOutMin=[]  SumOutMax=[]  SaturationOutMin=[]  SaturationOutMax=[]  PParamMin=[]  PParamMax=[]  IParamMin=[]  IParamMax=[]  DParamMin=[]  DParamMax=[]  NParamMin=[]  NParamMax=[]  KbParamMin=[]  KbParamMax=[]  KtParamMin=[]  KtParamMax=[]  KbOutMin=[]  KbOutMax=[]  KtOutMin=[]  KtOutMax=[]  IntegratorOutMin=[]  IntegratorOutMax=[]  FilterOutMin=[]  FilterOutMax=[]  SumI1OutMin=[]  SumI1OutMax=[]  SumI2OutMin=[]  SumI2OutMax=[]  SumI3OutMin=[]  SumI3OutMax=[]  SumI4OutMin=[]  SumI4OutMax=[]  SumDOutMin=[]  SumDOutMax=[]  DifferentiatorOutMin=[]  DifferentiatorOutMax=[]  FilterDiffOutCoefMin=[]  FilterDiffOutCoefMax=[]  ReciprocalOutMin=[]  ReciprocalOutMax=[]  SumDenOutMin=[]  SumDenOutMax=[]  SumNumOutMin=[]  SumNumOutMax=[]  DivideOutMin=[]  DivideOutMax=[]  UdiffTsProdOutMin=[]  UdiffTsProdOutMax=[]  NTsProdOutMin=[]  NTsProdOutMax=[]  UintegralTsProdOutMin=[]  UintegralTsProdOutMax=[]  UngainTsProdOutMin=[]  UngainTsProdOutMax=[]  ClampingZeroOutDataTypeStr=Inherit: Inherit via back propagation  ClampingZeroOutMin=[]  ClampingZeroOutMax=[]  FilterDenConstantOutDataTypeStr=Inherit: Inherit via back propagation  FilterDenConstantOutMin=[]  FilterDenConstantOutMax=[]  PCopyOutDataTypeStr=Inherit: Inherit via back propagation  PCopyOutMin=[]  PCopyOutMax=[]  NCopyOutDataTypeStr=Inherit: Inherit via back propagation  NCopyOutMin=[]  NCopyOutMax=[]  IntegratorContinuousStateAttributes=''  IntegratorStateMustResolveToSignalObject=off  IntegratorRTWStateStorageClass=Auto  FilterContinuousStateAttributes=''  FilterStateMustResolveToSignalObject=off  FilterRTWStateStorageClass=Auto  ParallelPVariant=ExternalParameters  IdealPVariant=Disabled  IVariant=ExternalParameters  DVariant=ExternalParameters  IntegratorVariant=Discrete  SatVariant=External  AWVariant=DiscClampingParallel  PCopyVariant=Disabled  TRVariant=Disabled  FdbkBlocksVariant=Feedback  IdealPFdbkVariant=Passthrough  SatFdbkVariant=Passthrough  DerivativeFilterVariant=ForwardEulerFilter  NVariant=ExternalParameters  NCopyVariant=Disabled  FilterICVariant=InternalICsFilter  IntegratorICVariant=InternalICs  ExternalResetVariant=ExternalReset  TRSumVariant=Passthrough  SumFdbkVariant=Enabled  SumVariant=Sum_PID  TsampFilterVariant=InternalTs  TsampNgainVariant=Passthrough  TsampIntegralVariant=Passthrough  ExternalSaturationOutDataTypeStr=Inherit: Same as second input  aMode=0
  Subsystem : Subsystem
  Sum1 : Sum  Inputs=|+-
  velocity lookup : Constant  Value=velocity_lookup
  Control Effort 1 : Outport
  wires:
  Constant3/1 -> PID Controller/5
  Constant2/1 -> Subsystem/5(pid_kd)
  Constant1/1 -> Subsystem/4(pid_ki)
  Subsystem/3(Out3) -> PID Controller/4
  Subsystem/2(Out2) -> PID Controller/3
  Subsystem/1(Out1) -> PID Controller/2
  velocity lookup/1 -> Subsystem/3(velocity lookup)
  Constant/1 -> Subsystem/2(pid_kp)
  velocity/1 -> Subsystem/1(velocity)
  ResetSignal/1 -> PID Controller/6
  PID Controller/1 -> Control Effort 1/1
  l_lim/1 -> PID Controller/8
  modified slip ratio measurement/1 -> Sum1/2
  u_lim/1 -> PID Controller/7
  modified slip ratio reference/1 -> Sum1/1
  Sum1/1 -> PID Controller/1

== system TorqueVect/CarMaker/IPG Vehicle/PowerTrain/PTControl Example/PTControl_TV_MFE25/Full Control Loop/TC 3 ==
  modified slip ratio reference : Inport
  u_lim : Inport  Port=2
  modified slip ratio measurement : Inport  Port=3
  l_lim : Inport  Port=4
  ResetSignal : Inport  Port=5
  velocity : Inport  Port=6
  Constant : Constant  Value=kp
  Constant1 : Constant  Value=ki
  Constant2 : Constant  Value=kd
  Constant3 : Constant  Value=N
  PID Controller : slpidlib/PID Controller  Controller=PID  Form=Parallel  TimeDomain=Discrete-time  UseExternalTs=off  SampleTime=Ts  IntegratorMethod=Trapezoidal  FilterMethod=Forward Euler  ControllerParametersSource=external  P=kp  I=ki  UseKiTs=on  D=kd  N=100  UseFilter=on  TunerSelectOption=Transfer Function Based (PID Tuner App)  InitialConditionSource=internal  InitialConditionForIntegrator=0  InitialConditionForFilter=0  DifferentiatorICPrevScaledInput=0  ExternalReset=either  TrackingMode=off  Kt=1  LimitOutput=on  SatLimitsSource=external  UpperSaturationLimit=inf  LowerSaturationLimit=-inf  LinearizeAsGain=on  AntiWindupMode=clamping  Kb=1  POutMin=[]  POutMax=[]  IOutMin=[]  IOutMax=[]  DOutMin=[]  DOutMax=[]  NOutMin=[]  NOutMax=[]  SumOutMin=[]  SumOutMax=[]  SaturationOutMin=[]  SaturationOutMax=[]  PParamMin=[]  PParamMax=[]  IParamMin=[]  IParamMax=[]  DParamMin=[]  DParamMax=[]  NParamMin=[]  NParamMax=[]  KbParamMin=[]  KbParamMax=[]  KtParamMin=[]  KtParamMax=[]  KbOutMin=[]  KbOutMax=[]  KtOutMin=[]  KtOutMax=[]  IntegratorOutMin=[]  IntegratorOutMax=[]  FilterOutMin=[]  FilterOutMax=[]  SumI1OutMin=[]  SumI1OutMax=[]  SumI2OutMin=[]  SumI2OutMax=[]  SumI3OutMin=[]  SumI3OutMax=[]  SumI4OutMin=[]  SumI4OutMax=[]  SumDOutMin=[]  SumDOutMax=[]  DifferentiatorOutMin=[]  DifferentiatorOutMax=[]  FilterDiffOutCoefMin=[]  FilterDiffOutCoefMax=[]  ReciprocalOutMin=[]  ReciprocalOutMax=[]  SumDenOutMin=[]  SumDenOutMax=[]  SumNumOutMin=[]  SumNumOutMax=[]  DivideOutMin=[]  DivideOutMax=[]  UdiffTsProdOutMin=[]  UdiffTsProdOutMax=[]  NTsProdOutMin=[]  NTsProdOutMax=[]  UintegralTsProdOutMin=[]  UintegralTsProdOutMax=[]  UngainTsProdOutMin=[]  UngainTsProdOutMax=[]  ClampingZeroOutDataTypeStr=Inherit: Inherit via back propagation  ClampingZeroOutMin=[]  ClampingZeroOutMax=[]  FilterDenConstantOutDataTypeStr=Inherit: Inherit via back propagation  FilterDenConstantOutMin=[]  FilterDenConstantOutMax=[]  PCopyOutDataTypeStr=Inherit: Inherit via back propagation  PCopyOutMin=[]  PCopyOutMax=[]  NCopyOutDataTypeStr=Inherit: Inherit via back propagation  NCopyOutMin=[]  NCopyOutMax=[]  IntegratorContinuousStateAttributes=''  IntegratorStateMustResolveToSignalObject=off  IntegratorRTWStateStorageClass=Auto  FilterContinuousStateAttributes=''  FilterStateMustResolveToSignalObject=off  FilterRTWStateStorageClass=Auto  ParallelPVariant=ExternalParameters  IdealPVariant=Disabled  IVariant=ExternalParameters  DVariant=ExternalParameters  IntegratorVariant=Discrete  SatVariant=External  AWVariant=DiscClampingParallel  PCopyVariant=Disabled  TRVariant=Disabled  FdbkBlocksVariant=Feedback  IdealPFdbkVariant=Passthrough  SatFdbkVariant=Passthrough  DerivativeFilterVariant=ForwardEulerFilter  NVariant=ExternalParameters  NCopyVariant=Disabled  FilterICVariant=InternalICsFilter  IntegratorICVariant=InternalICs  ExternalResetVariant=ExternalReset  TRSumVariant=Passthrough  SumFdbkVariant=Enabled  SumVariant=Sum_PID  TsampFilterVariant=InternalTs  TsampNgainVariant=Passthrough  TsampIntegralVariant=Passthrough  ExternalSaturationOutDataTypeStr=Inherit: Same as second input  aMode=0
  Subsystem : Subsystem
  Sum1 : Sum  Inputs=|+-
  velocity lookup : Constant  Value=velocity_lookup
  Control Effort 1 : Outport
  wires:
  Constant3/1 -> PID Controller/5
  Constant2/1 -> Subsystem/5(pid_kd)
  Constant1/1 -> Subsystem/4(pid_ki)
  Subsystem/3(Out3) -> PID Controller/4
  Subsystem/2(Out2) -> PID Controller/3
  Subsystem/1(Out1) -> PID Controller/2
  velocity lookup/1 -> Subsystem/3(velocity lookup)
  Constant/1 -> Subsystem/2(pid_kp)
  velocity/1 -> Subsystem/1(velocity)
  ResetSignal/1 -> PID Controller/6
  PID Controller/1 -> Control Effort 1/1
  l_lim/1 -> PID Controller/8
  modified slip ratio measurement/1 -> Sum1/2
  u_lim/1 -> PID Controller/7
  modified slip ratio reference/1 -> Sum1/1
  Sum1/1 -> PID Controller/1

== system TorqueVect/CarMaker/IPG Vehicle/PowerTrain/PTControl Example/PTControl_TV_MFE25/Full Control Loop/TC 4 ==
  modified slip ratio reference : Inport
  u_lim : Inport  Port=2
  modified slip ratio measurement : Inport  Port=3
  l_lim : Inport  Port=4
  ResetSignal : Inport  Port=5
  velocity : Inport  Port=6
  Constant : Constant  Value=kp
  Constant1 : Constant  Value=ki
  Constant2 : Constant  Value=kd
  Constant3 : Constant  Value=N
  PID Controller : slpidlib/PID Controller  Controller=PID  Form=Parallel  TimeDomain=Discrete-time  UseExternalTs=off  SampleTime=Ts  IntegratorMethod=Trapezoidal  FilterMethod=Forward Euler  ControllerParametersSource=external  P=kp  I=ki  UseKiTs=on  D=kd  N=100  UseFilter=on  TunerSelectOption=Transfer Function Based (PID Tuner App)  InitialConditionSource=internal  InitialConditionForIntegrator=0  InitialConditionForFilter=0  DifferentiatorICPrevScaledInput=0  ExternalReset=either  TrackingMode=off  Kt=1  LimitOutput=on  SatLimitsSource=external  UpperSaturationLimit=inf  LowerSaturationLimit=-inf  LinearizeAsGain=on  AntiWindupMode=clamping  Kb=1  POutMin=[]  POutMax=[]  IOutMin=[]  IOutMax=[]  DOutMin=[]  DOutMax=[]  NOutMin=[]  NOutMax=[]  SumOutMin=[]  SumOutMax=[]  SaturationOutMin=[]  SaturationOutMax=[]  PParamMin=[]  PParamMax=[]  IParamMin=[]  IParamMax=[]  DParamMin=[]  DParamMax=[]  NParamMin=[]  NParamMax=[]  KbParamMin=[]  KbParamMax=[]  KtParamMin=[]  KtParamMax=[]  KbOutMin=[]  KbOutMax=[]  KtOutMin=[]  KtOutMax=[]  IntegratorOutMin=[]  IntegratorOutMax=[]  FilterOutMin=[]  FilterOutMax=[]  SumI1OutMin=[]  SumI1OutMax=[]  SumI2OutMin=[]  SumI2OutMax=[]  SumI3OutMin=[]  SumI3OutMax=[]  SumI4OutMin=[]  SumI4OutMax=[]  SumDOutMin=[]  SumDOutMax=[]  DifferentiatorOutMin=[]  DifferentiatorOutMax=[]  FilterDiffOutCoefMin=[]  FilterDiffOutCoefMax=[]  ReciprocalOutMin=[]  ReciprocalOutMax=[]  SumDenOutMin=[]  SumDenOutMax=[]  SumNumOutMin=[]  SumNumOutMax=[]  DivideOutMin=[]  DivideOutMax=[]  UdiffTsProdOutMin=[]  UdiffTsProdOutMax=[]  NTsProdOutMin=[]  NTsProdOutMax=[]  UintegralTsProdOutMin=[]  UintegralTsProdOutMax=[]  UngainTsProdOutMin=[]  UngainTsProdOutMax=[]  ClampingZeroOutDataTypeStr=Inherit: Inherit via back propagation  ClampingZeroOutMin=[]  ClampingZeroOutMax=[]  FilterDenConstantOutDataTypeStr=Inherit: Inherit via back propagation  FilterDenConstantOutMin=[]  FilterDenConstantOutMax=[]  PCopyOutDataTypeStr=Inherit: Inherit via back propagation  PCopyOutMin=[]  PCopyOutMax=[]  NCopyOutDataTypeStr=Inherit: Inherit via back propagation  NCopyOutMin=[]  NCopyOutMax=[]  IntegratorContinuousStateAttributes=''  IntegratorStateMustResolveToSignalObject=off  IntegratorRTWStateStorageClass=Auto  FilterContinuousStateAttributes=''  FilterStateMustResolveToSignalObject=off  FilterRTWStateStorageClass=Auto  ParallelPVariant=ExternalParameters  IdealPVariant=Disabled  IVariant=ExternalParameters  DVariant=ExternalParameters  IntegratorVariant=Discrete  SatVariant=External  AWVariant=DiscClampingParallel  PCopyVariant=Disabled  TRVariant=Disabled  FdbkBlocksVariant=Feedback  IdealPFdbkVariant=Passthrough  SatFdbkVariant=Passthrough  DerivativeFilterVariant=ForwardEulerFilter  NVariant=ExternalParameters  NCopyVariant=Disabled  FilterICVariant=InternalICsFilter  IntegratorICVariant=InternalICs  ExternalResetVariant=ExternalReset  TRSumVariant=Passthrough  SumFdbkVariant=Enabled  SumVariant=Sum_PID  TsampFilterVariant=InternalTs  TsampNgainVariant=Passthrough  TsampIntegralVariant=Passthrough  ExternalSaturationOutDataTypeStr=Inherit: Same as second input  aMode=0
  Subsystem : Subsystem
  Sum1 : Sum  Inputs=|+-
  velocity lookup : Constant  Value=velocity_lookup
  Control Effort 1 : Outport
  wires:
  Constant3/1 -> PID Controller/5
  Constant2/1 -> Subsystem/5(pid_kd)
  Constant1/1 -> Subsystem/4(pid_ki)
  Subsystem/3(Out3) -> PID Controller/4
  Subsystem/2(Out2) -> PID Controller/3
  Subsystem/1(Out1) -> PID Controller/2
  velocity lookup/1 -> Subsystem/3(velocity lookup)
  Constant/1 -> Subsystem/2(pid_kp)
  velocity/1 -> Subsystem/1(velocity)
  ResetSignal/1 -> PID Controller/6
  PID Controller/1 -> Control Effort 1/1
  l_lim/1 -> PID Controller/8
  modified slip ratio measurement/1 -> Sum1/2
  u_lim/1 -> PID Controller/7
  modified slip ratio reference/1 -> Sum1/1
  Sum1/1 -> PID Controller/1

== system TorqueVect/CarMaker/IPG Vehicle/PowerTrain/PTControl Example/PTControl_TV_MFE25/New TC/Reference Generator1 ==
  note: Modified slip ratio targets
  note: Vehicle velocity
  note: For throttle sign and Product:
      | If positive, normal reference
      | If negative (regen), similar reference but negative (negative target slip*times speed), this might need to change to account for regen limits
      | If 0, target zero
  x2 : Inport
  Front SR Target : Inport  Port=2
  Rear SR Target : Inport  Port=3
  Constant : Constant
  Product1 : Product
  Product2 : Product
  Switch : Switch  Criteria=u2 > Threshold  Threshold=1  SaturateOnIntegerOverflow=off  InputSameDT=off
  R1 : Outport
  L1 : Outport  Port=2
  R2 : Outport  Port=3
  L2 : Outport  Port=4
  wires:
  Front SR Target/1 -> Product1/1
  Product1/1 -> L1/1, R1/1
  Product2/1 -> L2/1, R2/1
  Rear SR Target/1 -> Product2/2
  Switch/1 -> Product2/1, Product1/2
  x2/1 -> Switch/1, Switch/2
  Constant/1 -> Switch/3
